simulink model "FullFMS_2026_02_18_V0_3_9"  (R2025b)
settings: Solver=ode23tb  StartTime=0.0  StopTime=inf  MaxStep=0.1  RelTol=1e-2
PreLoadFcn:
  | load("BUS_CONFIG.mat")
libraries: opcualib x8
(part 2 of 4)

== matlab function FullFMS_2026_02_18_V0_3_9/Feedback_80 ==
  data: u1 input; F_82_Pist_Adv output; u2 input; u3 input; u4 input; u5 input; u6 input; u7 input; u8 input; u9 input; u10 input; u11 input; u12 input; u13 input; F_82_Suction_On output; F_82_Suction_Off output; F_82_Arm_2_Del output; F_82_Arm_2_Mag output; F_83_Led_Start output; F_83_Led_Reset output; F_83_Led_Extra1 output; F_83_Led_Extra2 output; F_83_Panel_O4 output; F_83_Panel_O5 output; F_83_Panel_O6 output; F_83_Panel_O7 output
function [F_82_Pist_Adv,F_82_Suction_On,F_82_Suction_Off,F_82_Arm_2_Del, ...
    F_82_Arm_2_Mag,F_83_Led_Start,F_83_Led_Reset,F_83_Led_Extra1,...
    F_83_Led_Extra2,F_83_Panel_O4,F_83_Panel_O5,F_83_Panel_O6,...
    F_83_Panel_O7] = fcn_feedbacks(u1,u2,u3,u4,u5,u6,u7,u8,u9,...
    u10,u11,u12,u13)

F_82_Pist_Adv = u1;
F_82_Suction_On = u2;
F_82_Suction_Off = u3;
F_82_Arm_2_Del = u4;
F_82_Arm_2_Mag = u5;
F_83_Led_Start = u6;
F_83_Led_Reset = u7;
F_83_Led_Extra1 = u8;
F_83_Led_Extra2 = u9;
F_83_Panel_O4 = u10;
F_83_Panel_O5 = u11;
F_83_Panel_O6 = u12;
F_83_Panel_O7 = u13;

== matlab function FullFMS_2026_02_18_V0_3_9/Control_80 ==
  data: C_85_Initialization output; C_85_Part_Del output; C_85_Part_Mag output; C_86_Mag_Parts output; C_87_RQ_MParts output; u1 input; u2 input; u3 input; u4 input; u5 input; u6 input; u7 input; C_82_Profibus output; C_83_RQ_Parts output; C_85_Start output; C_85_Single output; C_85_Continuous output; C_85_Counted output; u8 input; u9 input; u10 input; u11 input
function [C_85_Initialization, C_85_Part_Del, C_85_Part_Mag, C_86_Mag_Parts,...
C_87_RQ_MParts, C_82_Profibus, C_83_RQ_Parts, C_85_Start, C_85_Single,...
C_85_Continuous, C_85_Counted]...
= fcn_controls(u1,u2,u3,u4,u5,u6,u7,u8,u9,u10,u11)

C_85_Initialization = u1;
C_85_Part_Del = u2;
C_85_Part_Mag = u3;
C_86_Mag_Parts = u4;
C_87_RQ_MParts = u5;
C_82_Profibus = u6;
C_83_RQ_Parts = u7;
C_85_Start = u8;
C_85_Single = u9;
C_85_Continuous = u10;
C_85_Counted = u11;

== matlab function FullFMS_2026_02_18_V0_3_9/AS-i_70 ==
  data: u1 input; A_74_Request output; u2 input; u3 input; u4 input; u5 input; u6 input; u7 input; u8 input; u9 input; A_74_No_Cart output; A_74_Cart_Full output; A_74_CRoute_Out output; A_74_CRoute_In80 output; A_73_TestCartID output double; A_74_Cart_Stat output; A_74_Cart_Next output; A_74_Optic output; A_74_Count output; A_74_Pist_Bck output; A_74_Release_FB output; A_74_CRoute_In output; u10 input; u11 input; u12 input; u13 input
function [A_74_Request, A_74_No_Cart, A_74_Cart_Full, A_74_CRoute_Out,...
    A_74_CRoute_In80, A_73_TestCartID, A_74_Cart_Stat, ...
          A_74_Cart_Next, A_74_Optic, A_74_Count, A_74_Pist_Bck, ...
          A_74_Release_FB,...
          A_74_CRoute_In] = fcn_Asi(u1, u2, u3, u4, u5, u6, u7, u8, u9,...
          u10, u11, u12, u13)

A_74_Request = u1;
A_74_No_Cart = u2;
A_74_Cart_Full = u3;
A_74_CRoute_Out = u4;
A_74_CRoute_In80 = u5;
A_73_TestCartID = u6;
A_74_Cart_Stat = u7;
A_74_Cart_Next = u8;
A_74_Optic = u9;
A_74_Count = u10;
A_74_Pist_Bck = u11;
A_74_Release_FB = u12;
A_74_CRoute_In = u13;

== matlab function FullFMS_2026_02_18_V0_3_9/Sensors_80 ==
  data: u1 input; u2 input; u3 input; u4 input; u5 input; u6 input; u7 input; u8 input; u9 input; u10 input; u11 input; u12 input; u13 input; u14 input; u15 input; O_80_Mag_Full output; O_80_Pist_Back output; O_80_Pist_Fwd output; O_80_Part_Stuck output; O_80_Arm_Mag output; O_80_Arm_Del output; O_80_Mag_Empty output; O_81_Start output; O_81_Stop output; O_81_Key_Pos output; O_81_Reset output; O_81_Panel_I4 output; O_81_Panel_I5 output; O_81_Panel_I6 output; O_81_Panel_I7 output
function [O_80_Mag_Full,O_80_Pist_Back,O_80_Pist_Fwd,O_80_Part_Stuck,...
    O_80_Arm_Mag,O_80_Arm_Del,O_80_Mag_Empty,O_81_Start,O_81_Stop,...
    O_81_Key_Pos,O_81_Reset,O_81_Panel_I4,O_81_Panel_I5,O_81_Panel_I6,...
    O_81_Panel_I7] = fcn_sensors(u1,u2,u3,u4,u5,u6,u7,u8,u9,...
    u10,u11,u12,u13,u14,u15)

O_80_Mag_Full = u1;
O_80_Pist_Back = u2;
O_80_Pist_Fwd = u3;
O_80_Part_Stuck = u4;
O_80_Arm_Mag = u5;
O_80_Arm_Del = u6;
O_80_Mag_Empty = u7;
O_81_Start = u8;
O_81_Stop = u9;
O_81_Key_Pos = u10;
O_81_Reset = u11;
O_81_Panel_I4 = u12;
O_81_Panel_I5 = u13;
O_81_Panel_I6 = u14;
O_81_Panel_I7 = u15;

== matlab function FullFMS_2026_02_18_V0_3_9/Control_70 ==
  data: C_75_Initialization output; C_75_ID_Delivery1 output; C_75_ID_Delivery2 output; C_75_Part_Del output; C_75_RQ_Part_Del output; C_75_RQ_Wrong output; C_75_Identified80 output; C_75_Requested80 output; u1 input; C_72_Profibus output; u2 input; u3 input; u4 input; u5 input; u6 input; u7 input; u8 input; u9 input; u10 input; u11 input; u12 input; u13 input; C_75_RQ_Delivery1 output; C_75_RQ_Delivery2 output; C_75_Identified output; C_75_Requested output
function [C_75_Initialization, C_75_ID_Delivery1, C_75_ID_Delivery2, ...
          C_75_Part_Del, C_75_RQ_Part_Del, C_75_RQ_Wrong, C_75_Identified80, ...
          C_75_Requested80, C_72_Profibus, C_75_RQ_Delivery1, C_75_RQ_Delivery2, C_75_Identified, ...
          C_75_Requested] = fcn_Control(u1, u2, u3, u4, u5, u6, u7, u8, u9, u10, u11, u12, u13)

C_75_Initialization = u1;
C_75_ID_Delivery1 = u2;
C_75_ID_Delivery2 = u3;
C_75_Part_Del = u4;
C_75_RQ_Part_Del = u5;
C_75_RQ_Wrong = u6;
C_75_Identified80 = u7;
C_75_Requested80 = u8;
C_72_Profibus = u9;
C_75_RQ_Delivery1 = u10;
C_75_RQ_Delivery2 = u11;
C_75_Identified = u12;
C_75_Requested = u13;

== matlab function FullFMS_2026_02_18_V0_3_9/Feedback_70 ==
  data: u1 input; F_72_Elev_Down output; u2 input; u3 input; u4 input; u5 input; u6 input; u7 input; u8 input; u9 input; u10 input; u11 input; u12 input; F_72_Elev_Up output; F_72_Eject_Part output; F_72_Air_On output; F_73_Led_Start output; F_73_Led_Reset output; F_73_Led_Extra1 output; F_73_Led_Extra2 output; F_73_Panel_O4 output; F_73_Panel_O5 output; F_73_Panel_O6 output; F_73_Panel_O7 output
function [F_72_Elev_Down, F_72_Elev_Up, F_72_Eject_Part, F_72_Air_On, ...
          F_73_Led_Start, F_73_Led_Reset, F_73_Led_Extra1, F_73_Led_Extra2, ...
          F_73_Panel_O4, F_73_Panel_O5, F_73_Panel_O6, F_73_Panel_O7] = ...
          fcn_Feedback(u1, u2, u3, u4, u5, u6, u7, u8, u9, u10, u11, u12)

F_72_Elev_Down = u1;
F_72_Elev_Up = u2;
F_72_Eject_Part = u3;
F_72_Air_On = u4;
F_73_Led_Start = u5;
F_73_Led_Reset = u6;
F_73_Led_Extra1 = u7;
F_73_Led_Extra2 = u8;
F_73_Panel_O4 = u9;
F_73_Panel_O5 = u10;
F_73_Panel_O6 = u11;
F_73_Panel_O7 = u12;

== matlab function FullFMS_2026_02_18_V0_3_9/Sensors_70 ==
  data: u1 input; O_70_SInductive output; u2 input; u3 input; u4 input; u5 input; u6 input; u7 input; u8 input; u9 input; u10 input; u11 input; u12 input; u13 input; u14 input; u15 input; O_70_SPart output; O_70_SStation output; O_70_SPart_Height output; O_70_Elev_High output; O_70_Elev_Low output; O_70_Pist_Back output; O_71_Start output; O_71_Stop output; O_71_Key_Pos output; O_71_Reset output; O_71_Panel_I4 output; O_71_Panel_I5 output; O_71_Panel_I6 output; O_71_Panel_I7 output
function [O_70_SInductive, O_70_SPart, O_70_SStation, O_70_SPart_Height, ...
          O_70_Elev_High, O_70_Elev_Low, O_70_Pist_Back, O_71_Start, ...
          O_71_Stop, O_71_Key_Pos, O_71_Reset, O_71_Panel_I4, O_71_Panel_I5, ...
          O_71_Panel_I6, O_71_Panel_I7] = ...
          fcn_Sensors(u1, u2, u3, u4, u5, u6, u7, u8, u9, u10, ...
          u11, u12, u13, u14, u15)

O_70_SInductive = u1;
O_70_SPart = u2;
O_70_SStation = u3;
O_70_SPart_Height = u4;
O_70_Elev_High = u5;
O_70_Elev_Low = u6;
O_70_Pist_Back = u7;
O_71_Start = u8;
O_71_Stop = u9;
O_71_Key_Pos = u10;
O_71_Reset = u11;
O_71_Panel_I4 = u12;
O_71_Panel_I5 = u13;
O_71_Panel_I6 = u14;
O_71_Panel_I7 = u15;
